simulink model "exampleUnipolar"  (R2018a)
settings: Solver=ode23tb  StartTime=0.0  StopTime=.1  MaxStep=10e-6  RelTol=1e-3
libraries: powerlib x10, simulink x2, powerlib_meascontrol x1
settings Model: Creator=ivank  LastModifiedBy=bw_
settings SolverCC: InitialStep=10e-8

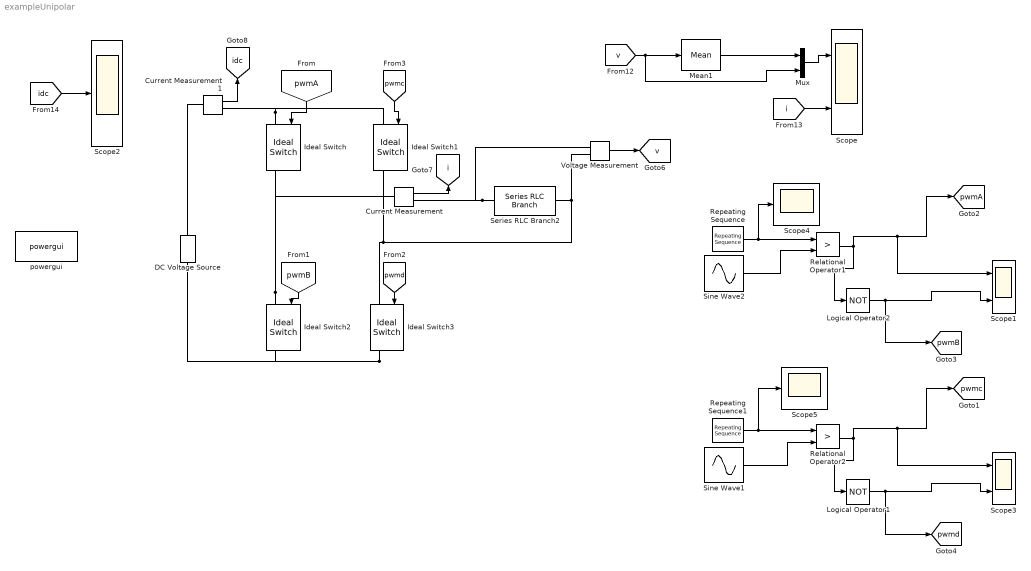
== system exampleUnipolar ==
  Current Measurement : powerlib/Measurements/Current Measurement  PhasorSimulation=off  OutputType=Complex  PSBequivalent=0
  Current Measurement1 : powerlib/Measurements/Current Measurement  PhasorSimulation=off  OutputType=Complex  PSBequivalent=0
  DC Voltage Source : powerlib/Electrical Sources/DC Voltage Source  Amplitude=100  Measurements=None
  Ideal Switch{,1..3} (4 alike) : powerlib/Power Electronics/Ideal Switch  Ron=0.001  Lon=0  IC=0  Rs=1e5  Cs=inf  Measurements=on
  Logical Operator1 : Logic  Operator=NOT  AllPortsSameDT=off  OutDataTypeStr=boolean
  Logical Operator2 : Logic  Operator=NOT  AllPortsSameDT=off  OutDataTypeStr=boolean
  Mean1 : powerlib_meascontrol/Measurements/Mean  Freq=1000  Vinit=0  Ts=0
  Mux : Mux  Inputs=2
  Relational Operator1 : RelationalOperator  Operator=>  OutDataTypeStr=boolean  RndMeth=Simplest
  Relational Operator2 : RelationalOperator  Operator=>  OutDataTypeStr=boolean  RndMeth=Simplest
  Repeating Sequence : simulink/Sources/Repeating Sequence  rep_seq_t=[0 1/4 3/4 1]*(1/1000)  rep_seq_y=[0 1 -1 0]
  Repeating Sequence1 : simulink/Sources/Repeating Sequence  rep_seq_t=[0 1/4 3/4 1]*(1/1000)  rep_seq_y=[0 1 -1 0]
  Scope : Scope  NumInputPorts=2
  Scope1 : Scope  NumInputPorts=2
  Scope2 : Scope
  Scope3 : Scope  NumInputPorts=2
  Scope4 : Scope
  Scope5 : Scope
  Series RLC Branch2 : powerlib/Elements/Series RLC Branch  LConnTagsString=__new0  RConnTagsString=__new0  BranchType=RL  Resistance=8  Inductance=5e-3  SetiL0=off  InitialCurrent=0  Capacitance=1e-6  Setx0=off  InitialVoltage=0  Measurements=None
  Sine Wave1 : Sin  Amplitude=0.1  Frequency=2*pi*50  Phase=pi  SampleTime=0
  Sine Wave2 : Sin  Amplitude=0.1  Frequency=2*pi*50  SampleTime=0
  Voltage Measurement : powerlib/Measurements/Voltage Measurement  PhasorSimulation=off  OutputType=Complex  PSBequivalent=0
  powergui : powerlib/powergui  Priority=1  SimulationMode=Continuous  SampleTime=50e-6  frequency=60  Iterations=50  frequencyindice=0  Pbase=100e6  ErrMax=1e-4  UnitsV=kV  UnitsW=MW  buscounter=0  FunctionMessages=off  echomessages=off  EnableUseOfTLC=off  CurrentSourceSwitches=off  DisableSnubberDevices=off  DisableRonSwitches=off  DisableVfSwitches=off  DisplayEquations=off  SolverType=Tustin/Backward Euler (TBE)  Interpol=off  ExternalGateDelay=off  methode=off  Ts=100  x0status=blocks  SPID=on  SwTol=0  HookPort=off  RestoreLinks=warning  ResistiveCurrentMeasurement=off  Frange=[0:2:500]  Ylog=off  Xlog=on  ShowGrid=off  save=off  variable=ZData  structure=v  ZoomFFT=off  StartTime=0.0  cycles=4  DisplayStyle=1  fundamental=50  FreqAxis=off  MaxFrequency=1000  frequencyindicesteady=1  RmsSteady=1  display=off
  tag scope: i=global, idc=global, pwmA=global, pwmB=global, pwmc=global, pwmd=global, v=global
  wires:
  [pwmc] -> Ideal Switch1/1
  Current Measurement/1 -> [i]
  [idc] -> Scope2/1
  Repeating Sequence/1 -> Scope4/1, Relational Operator1/1
  Relational Operator1/1 -> Scope1/1, [pwmA], Logical Operator2/1
  [v] -> Mux/2, Mean1/1
  Voltage Measurement/1 -> [v]
  [pwmd] -> Ideal Switch3/1
  Logical Operator2/1 -> [pwmB], Scope1/2
  [pwmA] -> Ideal Switch/1
  [pwmB] -> Ideal Switch2/1
  Current Measurement1/1 -> [idc]
  [i] -> Scope/2
  Logical Operator1/1 -> Scope3/2, [pwmd]
  Relational Operator2/1 -> Logical Operator1/1, [pwmc], Scope3/1
  Repeating Sequence1/1 -> Relational Operator2/1, Scope5/1
  Mean1/1 -> Mux/1
  Mux/1 -> Scope/1
  Sine Wave2/1 -> Relational Operator1/2
  Sine Wave1/1 -> Relational Operator2/2
  connections:
  Series RLC Branch2/RConn1 -- Voltage Measurement/LConn2 -- Ideal Switch1/RConn1 -- Ideal Switch3/LConn1
  Series RLC Branch2/LConn1 -- Voltage Measurement/LConn1 -- Current Measurement/RConn1
  Ideal Switch3/RConn1 -- Ideal Switch2/RConn1 -- DC Voltage Source/LConn1
  Ideal Switch2/LConn1 -- Ideal Switch/RConn1 -- Current Measurement/LConn1
  Ideal Switch/LConn1 -- Ideal Switch1/LConn1 -- Current Measurement1/RConn1
  DC Voltage Source/RConn1 -- Current Measurement1/LConn1
